simulink model "sampleModel156"  (R2021b)
settings: Solver=VariableStepAuto  StartTime=0.0  StopTime=10.0  RelTol=1e-3
undefined symbols (not defined in the file or in its folder): DiscIntNeverNeededParam, Newton, Raphson
libraries: simulink x12, slpidlib x2
settings Model: Creator=user  LastModifiedBy=user

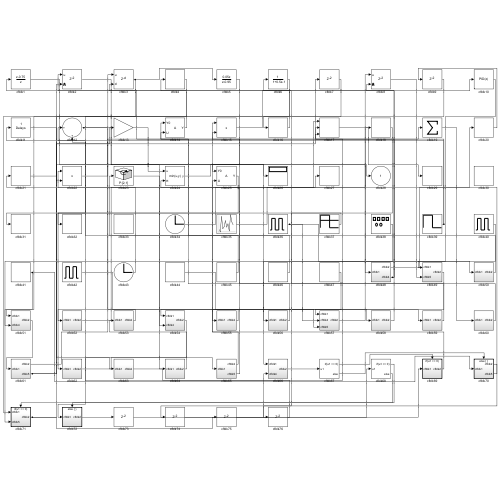
[thumbnail: Simulink's stored preview of the top-level diagram]
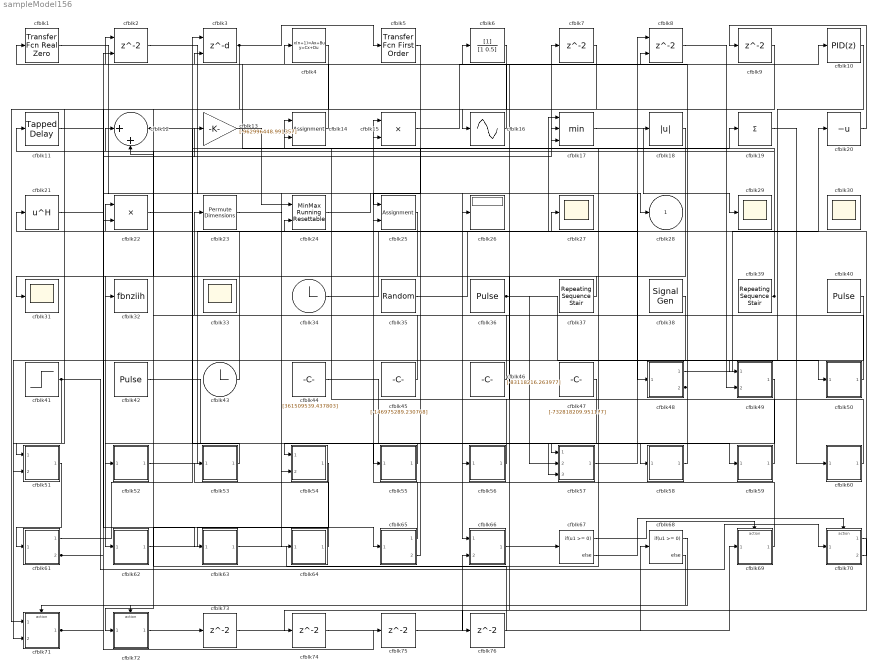
== system sampleModel156 ==
  cfblk1 : simulink/Discrete/Transfer Fcn Real Zero  ZeroZ=0.75  ICPrevInput=0.0  DoSatur=off
      settings: SourceProductBaseCode=SL
  cfblk10 : slpidlib/PID Controller  Controller=PID  Form=Parallel  TimeDomain=Discrete-time  UseExternalTs=off  SampleTime=1  IntegratorMethod=Forward Euler  FilterMethod=Forward Euler  ControllerParametersSource=internal  P=1  I=1  D=0  UseFilter=on  N=100  TunerSelectOption=Transfer Function Based (PID Tuner App)  InitialConditionSource=internal  InitialConditionForIntegrator=0  InitialConditionForFilter=0  DifferentiatorICPrevScaledInput=0  ExternalReset=none  TrackingMode=off  Kt=1  LimitOutput=off  SatLimitsSource=internal  UpperSaturationLimit=inf  LowerSaturationLimit=-inf  LinearizeAsGain=off  AntiWindupMode=none  Kb=1  POutMin=[]  POutMax=[]  IOutMin=[]  IOutMax=[]  DOutMin=[]  DOutMax=[]  NOutMin=[]  NOutMax=[]  SumOutMin=[]  SumOutMax=[]  SaturationOutMin=[]  SaturationOutMax=[]  PParamMin=[]  PParamMax=[]  IParamMin=[]  IParamMax=[]  DParamMin=[]  DParamMax=[]  NParamMin=[]  NParamMax=[]  KbParamMin=[]  KbParamMax=[]  KtParamMin=[]  KtParamMax=[]  KbOutMin=[]  KbOutMax=[]  KtOutMin=[]  KtOutMax=[]  IntegratorOutMin=[]  IntegratorOutMax=[]  FilterOutMin=[]  FilterOutMax=[]  SumI1OutMin=[]  SumI1OutMax=[]  SumI2OutMin=[]  SumI2OutMax=[]  SumI3OutMin=[]  SumI3OutMax=[]  SumI4OutMin=[]  SumI4OutMax=[]  SumDOutMin=[]  SumDOutMax=[]  DifferentiatorOutMin=[]  DifferentiatorOutMax=[]  FilterDiffOutCoefMin=[]  FilterDiffOutCoefMax=[]  ReciprocalOutMin=[]  ReciprocalOutMax=[]  SumDenOutMin=[]  SumDenOutMax=[]  SumNumOutMin=[]  SumNumOutMax=[]  DivideOutMin=[]  DivideOutMax=[]  UdiffTsProdOutMin=[]  UdiffTsProdOutMax=[]  NTsProdOutMin=[]  NTsProdOutMax=[]  UintegralTsProdOutMin=[]  UintegralTsProdOutMax=[]  UngainTsProdOutMin=[]  UngainTsProdOutMax=[]  IntegratorContinuousStateAttributes=''  IntegratorStateMustResolveToSignalObject=off  IntegratorRTWStateStorageClass=Auto  FilterContinuousStateAttributes=''  FilterStateMustResolveToSignalObject=off  FilterRTWStateStorageClass=Auto  ParallelPVariant=InternalParameters  IdealPVariant=Disabled  IVariant=InternalParameters  DVariant=InternalParameters  IntegratorVariant=Discrete  SatVariant=Disabled  AWVariant=Passthrough  PCopyVariant=Disabled  TRVariant=Disabled  FdbkBlocksVariant=Forward  IdealPFdbkVariant=Disabled  SatFdbkVariant=Disabled  DerivativeFilterVariant=ForwardEulerFilter  NVariant=InternalParameters  NCopyVariant=Disabled  FilterICVariant=InternalICsFilter  IntegratorICVariant=InternalICs  ExternalResetVariant=Disabled  TRSumVariant=Passthrough  SumFdbkVariant=Disabled  SumVariant=Sum_PID  TsampFilterVariant=InternalTs  TsampNgainVariant=Passthrough  TsampIntegralVariant=Passthrough  ExternalSaturationOutDataTypeStr=Inherit: Same as second input
  cfblk11 : simulink/Discrete/Tapped Delay  vinit=0.0  samptime=-1  NumDelays=1  DelayOrder=Oldest  includeCurrent=off
  cfblk12 : Sum  Inputs=|++
  cfblk13 : Gain  Gain=[-962996448.991357]
  cfblk14 : Assignment  DiagnosticForDimensions=Warning  IndexOptions=Index vector (dialog)  Indices=1  OutputSizes=1
  cfblk15 : Product  Inputs=**
  cfblk16 : Sin  TimeSource=Use external signal  SampleTime=0
  cfblk17 : MinMax  Inputs=3
  cfblk18 : Abs
  cfblk19 : Sum  Inputs=+
  cfblk2 : Delay  ShowEnablePort=on  SampleTime=1
      settings: InputPortMap=u0,e6
  cfblk20 : UnaryMinus
  cfblk21 : Math  Operator=hermitian  SaturateOnIntegerOverflow=on
  cfblk22 : Product
  cfblk23 : PermuteDimensions
  cfblk24 : simulink/Math Operations/MinMax Running Resettable  Function=min  vinit=0.0
  cfblk25 : Assignment  DiagnosticForDimensions=Warning  IndexOptions=Index vector (dialog)  Indices=1  OutputSizes=1
  cfblk26 : Display
  cfblk{27,29..31,33} (5 alike) : Scope
      cfblk30 settings: Floating=on
      cfblk33 settings: Floating=on
  cfblk3 : Delay  DelayLengthSource=Input port  SampleTime=1
      settings: InputPortMap=u0,p1
  cfblk32 : ToWorkspace  VariableName=fbnziih  SaveFormat=Timeseries  SampleTime=-1
  cfblk34 : Clock
  cfblk35 : UniformRandomNumber  Minimum=[-899286631.365557]  Maximum=[926374637.674813]  Seed=[29961251.000000]  SampleTime=0.1
  cfblk36 : DiscretePulseGenerator  PulseType=Time based  Amplitude=[-229932687.777880]  Period=[45551457.164221]  PulseWidth=5  PhaseDelay=[1.000000]
  cfblk37 : simulink/Sources/Repeating Sequence Stair  OutValues=[272091516.353895, -383976291.141123]  tsamp=-1  OutMin=[]  OutMax=[]  OutDataTypeStr=double  OutputDataTypeScalingMode=double  OutDataType=fixdt(0,8)  ConRadixGroup=Best Precision: Vector-wise  OutScaling=2^-12
  cfblk38 : SignalGenerator  WaveForm=sawtooth  Amplitude=[754582492.273324]
  cfblk39 : simulink/Sources/Repeating Sequence Stair  OutValues=[148032114.325394, 77359554.602000]  tsamp=-1  OutMin=[]  OutMax=[]  OutDataTypeStr=double  OutputDataTypeScalingMode=double  OutDataType=fixdt(0,8)  ConRadixGroup=Best Precision: Vector-wise  OutScaling=2^-12
  cfblk4 : DiscreteStateSpace
  cfblk40 : DiscretePulseGenerator  PulseType=Time based  Amplitude=[574486039.532884]  Period=[50865221.708180]  PulseWidth=5  PhaseDelay=[9.000000]
  cfblk41 : Step  Time=[32.000000]  Before=[271111049.835422]  After=[727022532.262540]  SampleTime=0
  cfblk42 : DiscretePulseGenerator  PulseType=Time based  Amplitude=[-857152997.487512]  Period=[21737191.178487]  PulseWidth=5  PhaseDelay=[9.000000]
  cfblk43 : Clock
  cfblk44 : Constant  Value=[361509539.437803]  SampleTime=1
  cfblk45 : Constant  Value=[-146975289.230768]  SampleTime=1
  cfblk46 : Constant  Value=[-83118216.263977]  SampleTime=1
  cfblk47 : Constant  Value=[-732818209.951177]  SampleTime=1
  cfblk48 : Subsystem
  cfblk49 : Subsystem
  cfblk5 : simulink/Discrete/Transfer Fcn First Order  PoleZ=0.95  ICPrevOutput=0.0  DoSatur=off
  cfblk50 : Subsystem
  cfblk51 : Subsystem
  cfblk52 : Subsystem
  cfblk53 : Subsystem
  cfblk54 : Subsystem
  cfblk55 : Subsystem
  cfblk56 : Subsystem
  cfblk57 : Subsystem
  cfblk58 : Subsystem
  cfblk59 : Subsystem
  cfblk6 : DiscreteFilter  SampleTime=1
  cfblk60 : Subsystem
  cfblk61 : Subsystem
  cfblk62 : Subsystem
  cfblk63 : Subsystem
  cfblk64 : Subsystem
  cfblk65 : Subsystem
  cfblk66 : Subsystem
  cfblk67 : If  IfExpression=u1 >= 0  SampleTime=1
  cfblk68 : If  IfExpression=u1 >= 0  SampleTime=1
  cfblk69 : Subsystem  TreatAsAtomicUnit=on
  cfblk{7,9,73..76} (6 alike) : Delay  SampleTime=1
  cfblk70 : Subsystem  TreatAsAtomicUnit=on
  cfblk71 : Subsystem  TreatAsAtomicUnit=on
  cfblk72 : Subsystem  TreatAsAtomicUnit=on
  cfblk8 : Delay  ShowEnablePort=on  SampleTime=1
      settings: InputPortMap=u0,e6
  cfblk28 : Outport
  wires:
  cfblk65/1(cfblk2) -> cfblk15/1
  cfblk13/1 -> cfblk24/1
  cfblk43/1 -> cfblk22/1
  cfblk51/1(cfblk2) -> cfblk61/1(cfblk1)
  cfblk37/1 -> cfblk31/1
  cfblk17/1 -> cfblk29/1
  cfblk46/1 -> cfblk23/1
  cfblk19/1 -> cfblk60/1(cfblk1)
  cfblk63/1(cfblk2) -> cfblk7/1
  cfblk66/1(cfblk2) -> cfblk67/1
  cfblk22/1 -> cfblk19/1
  cfblk6/1 -> cfblk71/1(cfblk1)
  cfblk48/1(cfblk2) -> cfblk20/1
  cfblk47/1 -> cfblk57/1(cfblk1)
  cfblk2/1 -> cfblk66/1(cfblk1)
  cfblk1/1 -> cfblk64/1(cfblk1)
  cfblk14/1 -> cfblk2/1
  cfblk25/1 -> cfblk62/1(cfblk1)
  cfblk5/1 -> cfblk25/1
  cfblk9/1 -> cfblk16/1
  cfblk65/2(cfblk5) -> cfblk24/2
  cfblk40/1 -> cfblk56/1(cfblk1)
  cfblk39/1 -> cfblk11/1, cfblk3/2
  cfblk36/1 -> cfblk50/1(cfblk1), cfblk57/2(cfblk4)
  cfblk45/1 -> cfblk12/1
  cfblk62/1(cfblk2) -> cfblk65/1(cfblk1)
  cfblk53/1(cfblk2) -> cfblk52/1(cfblk1)
  cfblk38/1 -> cfblk71/2(cfblk5)
  cfblk42/1 -> cfblk58/1(cfblk1)
  cfblk41/1 -> cfblk70/1(cfblk1), cfblk51/2(cfblk4)
  cfblk7/1 -> cfblk51/1(cfblk1)
  cfblk57/1(cfblk2) -> cfblk18/1
  cfblk56/1(cfblk2) -> cfblk14/1
  cfblk3/1 -> cfblk22/2, cfblk5/1
  cfblk35/1 -> cfblk8/1
  cfblk52/1(cfblk2) -> cfblk27/1
  cfblk44/1 -> cfblk59/1(cfblk1)
  cfblk58/1(cfblk2) -> cfblk8/2
  cfblk55/1(cfblk2) -> cfblk54/1(cfblk1)
  cfblk69/1(cfblk2) -> cfblk25/2
  cfblk21/1 -> cfblk26/1
  cfblk59/1(cfblk2) -> cfblk15/2
  cfblk70/2(cfblk5) -> cfblk21/1
  cfblk23/1 -> cfblk54/2(cfblk4)
  cfblk71/1(cfblk2) -> cfblk2/2, cfblk75/1
  cfblk24/1 -> cfblk28/1
  cfblk12/1 -> cfblk48/1(cfblk1), cfblk57/3(cfblk5)
  cfblk15/1 -> cfblk10/1
  cfblk48/2(cfblk4) -> cfblk4/1, cfblk17/3
  cfblk49/1(cfblk2) -> cfblk55/1(cfblk1)
  cfblk61/1(cfblk2) -> cfblk3/1
  cfblk60/1(cfblk2) -> cfblk6/1
  cfblk10/1 -> cfblk49/1(cfblk1)
  cfblk50/1(cfblk2) -> cfblk14/2
  cfblk11/1 -> cfblk63/1(cfblk1)
  cfblk4/1 -> cfblk32/1
  cfblk61/2(cfblk5) -> cfblk13/1, cfblk17/2
  cfblk34/1 -> cfblk17/1
  cfblk20/1 -> cfblk9/1
  cfblk64/1(cfblk2) -> cfblk53/1(cfblk1)
  cfblk54/1(cfblk2) -> cfblk72/1(cfblk1)
  cfblk8/1 -> cfblk49/2(cfblk5)
  cfblk16/1 -> cfblk1/1
  cfblk67/1 -> cfblk69/Action
  cfblk67/2 -> cfblk70/Action
  cfblk68/1 -> cfblk71/Action
  cfblk68/2 -> cfblk72/Action
  cfblk72/1(cfblk2) -> cfblk73/1
  cfblk73/1 -> cfblk69/1(cfblk1)
  cfblk70/1(cfblk2) -> cfblk74/1
  cfblk74/1 -> cfblk66/2(cfblk4)
  cfblk75/1 -> cfblk68/1
  cfblk18/1 -> cfblk76/1
  cfblk76/1 -> cfblk12/2

== system sampleModel156/cfblk48 ==
  cfblk1 : Inport
  cfblk3 : Bias  Bias=[-28596696.417519]
  cfblk2 : Outport
  cfblk4 : Outport  Port=2
  wires:
  cfblk1/1 -> cfblk3/1
  cfblk3/1 -> cfblk2/1, cfblk4/1

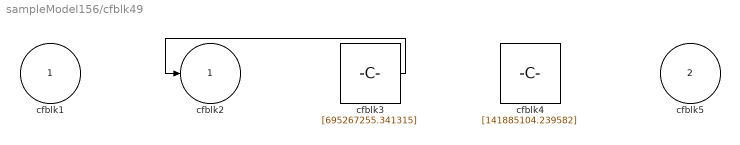
== system sampleModel156/cfblk49 ==
  cfblk1 : Inport
  cfblk5 : Inport  Port=2
  cfblk3 : Constant  Value=[695267255.341315]  SampleTime=1
  cfblk4 : Constant  Value=[141885104.239582]  SampleTime=1
  cfblk2 : Outport
  wires:
  cfblk3/1 -> cfblk2/1

== system sampleModel156/cfblk50 ==
  cfblk1 : Inport
  cfblk3 : Bias  Bias=[731161692.289361]
  cfblk2 : Outport
  wires:
  cfblk1/1 -> cfblk3/1
  cfblk3/1 -> cfblk2/1

== system sampleModel156/cfblk51 ==
  cfblk1 : Inport
  cfblk4 : Inport  Port=2
  cfblk3 : DiscreteFilter  SampleTime=1
  cfblk2 : Outport
  wires:
  cfblk4/1 -> cfblk2/1
  cfblk1/1 -> cfblk3/1

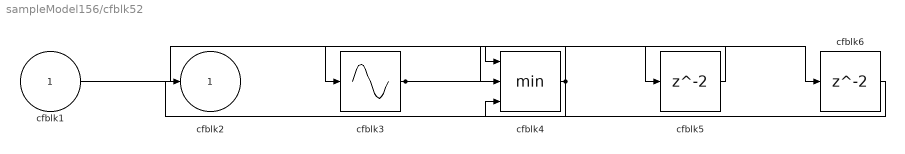
== system sampleModel156/cfblk52 ==
  cfblk1 : Inport
  cfblk3 : Sin  TimeSource=Use external signal  SampleTime=0
  cfblk4 : MinMax  Inputs=3
  cfblk5 : Delay  SampleTime=1
  cfblk6 : Delay  SampleTime=1
  cfblk2 : Outport
  wires:
  cfblk1/1 -> cfblk4/1
  cfblk3/1 -> cfblk5/1, cfblk6/1
  cfblk4/1 -> cfblk2/1, cfblk3/1
  cfblk5/1 -> cfblk4/2
  cfblk6/1 -> cfblk4/3

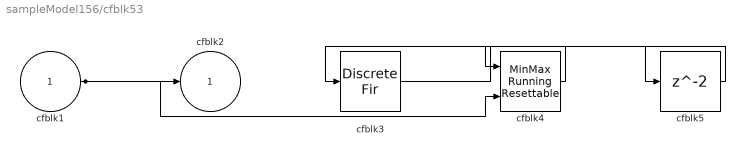
== system sampleModel156/cfblk53 ==
  cfblk1 : Inport
  cfblk3 : DiscreteFir  SampleTime=1
  cfblk4 : simulink/Math Operations/MinMax Running Resettable  Function=min  vinit=0.0
  cfblk5 : Delay  SampleTime=1
  cfblk2 : Outport
  wires:
  cfblk1/1 -> cfblk2/1, cfblk4/2
  cfblk4/1 -> cfblk3/1
  cfblk3/1 -> cfblk5/1
  cfblk5/1 -> cfblk4/1

== system sampleModel156/cfblk54 ==
  cfblk1 : Inport
  cfblk4 : Inport  Port=2
  cfblk3 : Product  Inputs=**
  cfblk2 : Outport
  wires:
  cfblk4/1 -> cfblk3/1
  cfblk1/1 -> cfblk3/2
  cfblk3/1 -> cfblk2/1

== system sampleModel156/cfblk55 ==
  cfblk1 : Inport
  cfblk3 : UnitDelay  HasFrameUpgradeWarning=on
  cfblk4 : Constant  Value=[458405676.200662]  SampleTime=1
  cfblk2 : Outport
  wires:
  cfblk1/1 -> cfblk3/1
  cfblk3/1 -> cfblk2/1

== system sampleModel156/cfblk56 ==
  cfblk1 : Inport
  cfblk3 : Sum  Inputs=+-
  cfblk4 : ComplexToMagnitudeAngle
  cfblk2 : Outport
  wires:
  cfblk4/1 -> cfblk3/1
  cfblk3/1 -> cfblk2/1
  cfblk4/2 -> cfblk3/2
  cfblk1/1 -> cfblk4/1

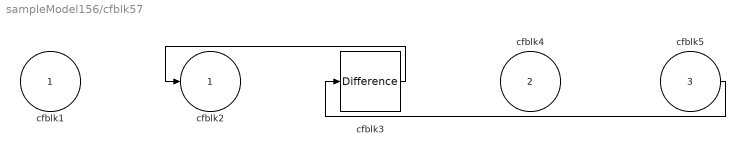
== system sampleModel156/cfblk57 ==
  cfblk1 : Inport
  cfblk4 : Inport  Port=2
  cfblk5 : Inport  Port=3
  cfblk3 : simulink/Discrete/Difference  ICPrevInput=0.0  OutMin=[]  OutMax=[]  OutDataTypeStr=Inherit: Inherit via back propagation  OutDataType=fixdt(1, 16)  OutScaling=2^-10  DoSatur=off
  cfblk2 : Outport
  wires:
  cfblk3/1 -> cfblk2/1
  cfblk5/1 -> cfblk3/1

== system sampleModel156/cfblk58 ==
  cfblk1 : Inport
  cfblk3 : DotProduct  InputSameDT=on  OutDataTypeStr=Inherit: Inherit via internal rule
  cfblk2 : Outport
  wires:
  cfblk1/1 -> cfblk3/1, cfblk3/2
  cfblk3/1 -> cfblk2/1

== system sampleModel156/cfblk59 ==
  cfblk1 : Inport
  cfblk3 : DiscreteStateSpace
  cfblk4 : simulink/Discrete/Transfer Fcn Lead or Lag  PoleZ=0.95  ZeroZ=0.75  ICPrevOutput=0.0  ICPrevInput=0.0  DoSatur=off
      settings: SourceProductBaseCode=SL
  cfblk2 : Outport
  wires:
  cfblk4/1 -> cfblk2/1
  cfblk1/1 -> cfblk3/1
  cfblk3/1 -> cfblk4/1

== system sampleModel156/cfblk60 ==
  cfblk1 : Inport
  cfblk3 : simulink/Discrete/Difference  ICPrevInput=0.0  OutMin=[]  OutMax=[]  OutDataTypeStr=Inherit: Inherit via back propagation  OutDataType=fixdt(1, 16)  OutScaling=2^-10  DoSatur=off
  cfblk4 : Squeeze
  cfblk2 : Outport
  wires:
  cfblk1/1 -> cfblk3/1
  cfblk3/1 -> cfblk4/1
  cfblk4/1 -> cfblk2/1

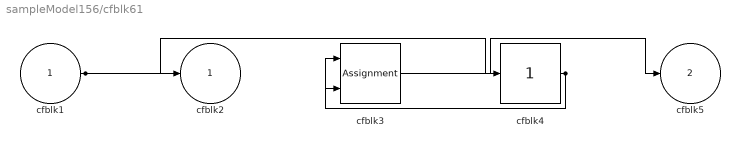
== system sampleModel156/cfblk61 ==
  cfblk1 : Inport
  cfblk3 : Assignment  DiagnosticForDimensions=Warning  IndexOptions=Index vector (dialog)  Indices=1  OutputSizes=1
  cfblk4 : simulink/Math Operations/Slider Gain  gain=1  low=0  high=2
  cfblk2 : Outport
  cfblk5 : Outport  Port=2
  wires:
  cfblk3/1 -> cfblk5/1
  cfblk1/1 -> cfblk2/1, cfblk4/1
  cfblk4/1 -> cfblk3/1, cfblk3/2

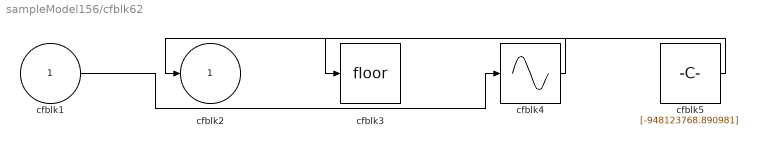
== system sampleModel156/cfblk62 ==
  cfblk1 : Inport
  cfblk3 : Rounding
  cfblk4 : Sin  TimeSource=Use external signal  SampleTime=0
  cfblk5 : Constant  Value=[-948123768.890981]  SampleTime=1
  cfblk2 : Outport
  wires:
  cfblk4/1 -> cfblk2/1
  cfblk1/1 -> cfblk4/1
  cfblk5/1 -> cfblk3/1

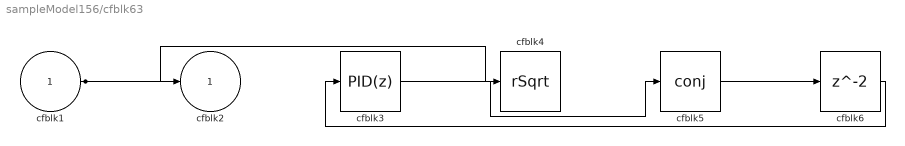
== system sampleModel156/cfblk63 ==
  cfblk1 : Inport
  cfblk3 : slpidlib/PID Controller  Controller=PID  Form=Parallel  TimeDomain=Discrete-time  UseExternalTs=off  SampleTime=1  IntegratorMethod=Forward Euler  FilterMethod=Forward Euler  ControllerParametersSource=internal  P=1  I=1  D=0  UseFilter=on  N=100  TunerSelectOption=Transfer Function Based (PID Tuner App)  InitialConditionSource=internal  InitialConditionForIntegrator=0  InitialConditionForFilter=0  DifferentiatorICPrevScaledInput=0  ExternalReset=none  TrackingMode=off  Kt=1  LimitOutput=off  SatLimitsSource=internal  UpperSaturationLimit=inf  LowerSaturationLimit=-inf  LinearizeAsGain=off  AntiWindupMode=none  Kb=1  POutMin=[]  POutMax=[]  IOutMin=[]  IOutMax=[]  DOutMin=[]  DOutMax=[]  NOutMin=[]  NOutMax=[]  SumOutMin=[]  SumOutMax=[]  SaturationOutMin=[]  SaturationOutMax=[]  PParamMin=[]  PParamMax=[]  IParamMin=[]  IParamMax=[]  DParamMin=[]  DParamMax=[]  NParamMin=[]  NParamMax=[]  KbParamMin=[]  KbParamMax=[]  KtParamMin=[]  KtParamMax=[]  KbOutMin=[]  KbOutMax=[]  KtOutMin=[]  KtOutMax=[]  IntegratorOutMin=[]  IntegratorOutMax=[]  FilterOutMin=[]  FilterOutMax=[]  SumI1OutMin=[]  SumI1OutMax=[]  SumI2OutMin=[]  SumI2OutMax=[]  SumI3OutMin=[]  SumI3OutMax=[]  SumI4OutMin=[]  SumI4OutMax=[]  SumDOutMin=[]  SumDOutMax=[]  DifferentiatorOutMin=[]  DifferentiatorOutMax=[]  FilterDiffOutCoefMin=[]  FilterDiffOutCoefMax=[]  ReciprocalOutMin=[]  ReciprocalOutMax=[]  SumDenOutMin=[]  SumDenOutMax=[]  SumNumOutMin=[]  SumNumOutMax=[]  DivideOutMin=[]  DivideOutMax=[]  UdiffTsProdOutMin=[]  UdiffTsProdOutMax=[]  NTsProdOutMin=[]  NTsProdOutMax=[]  UintegralTsProdOutMin=[]  UintegralTsProdOutMax=[]  UngainTsProdOutMin=[]  UngainTsProdOutMax=[]  IntegratorContinuousStateAttributes=''  IntegratorStateMustResolveToSignalObject=off  IntegratorRTWStateStorageClass=Auto  FilterContinuousStateAttributes=''  FilterStateMustResolveToSignalObject=off  FilterRTWStateStorageClass=Auto  ParallelPVariant=InternalParameters  IdealPVariant=Disabled  IVariant=InternalParameters  DVariant=InternalParameters  IntegratorVariant=Discrete  SatVariant=Disabled  AWVariant=Passthrough  PCopyVariant=Disabled  TRVariant=Disabled  FdbkBlocksVariant=Forward  IdealPFdbkVariant=Disabled  SatFdbkVariant=Disabled  DerivativeFilterVariant=ForwardEulerFilter  NVariant=InternalParameters  NCopyVariant=Disabled  FilterICVariant=InternalICsFilter  IntegratorICVariant=InternalICs  ExternalResetVariant=Disabled  TRSumVariant=Passthrough  SumFdbkVariant=Disabled  SumVariant=Sum_PID  TsampFilterVariant=InternalTs  TsampNgainVariant=Passthrough  TsampIntegralVariant=Passthrough  ExternalSaturationOutDataTypeStr=Inherit: Same as second input
  cfblk4 : Sqrt  Operator=rSqrt  AlgorithmType=Newton-Raphson  SaturateOnIntegerOverflow=on
  cfblk5 : Math  Operator=conj  SaturateOnIntegerOverflow=on
  cfblk6 : Delay  SampleTime=1
  cfblk2 : Outport
  wires:
  cfblk1/1 -> cfblk2/1, cfblk4/1
  cfblk3/1 -> cfblk5/1
  cfblk5/1 -> cfblk6/1
  cfblk6/1 -> cfblk3/1

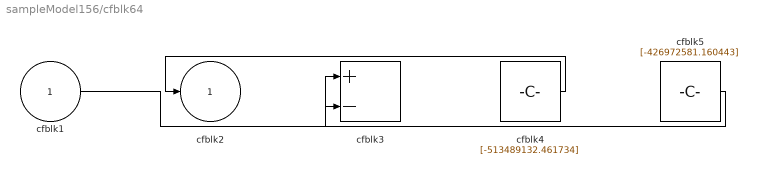
== system sampleModel156/cfblk64 ==
  cfblk1 : Inport
  cfblk3 : Sum  Inputs=+-
  cfblk4 : Constant  Value=[-513489132.461734]  SampleTime=1
  cfblk5 : Constant  Value=[-426972581.160443]  SampleTime=1
  cfblk2 : Outport
  wires:
  cfblk4/1 -> cfblk2/1
  cfblk5/1 -> cfblk3/1
  cfblk1/1 -> cfblk3/2

== system sampleModel156/cfblk65 ==
  cfblk1 : Inport
  cfblk3 : Reshape
  cfblk4 : Sum  Inputs=+
  cfblk2 : Outport
  cfblk5 : Outport  Port=2
  wires:
  cfblk4/1 -> cfblk3/1
  cfblk3/1 -> cfblk5/1
  cfblk1/1 -> cfblk2/1, cfblk4/1

== system sampleModel156/cfblk66 ==
  cfblk1 : Inport
  cfblk4 : Inport  Port=2
  cfblk3 : MinMax
  cfblk2 : Outport
  wires:
  cfblk1/1 -> cfblk3/1
  cfblk4/1 -> cfblk2/1

== system sampleModel156/cfblk69 ==
  cfblk1 : Inport
  Action Port : ActionPort  ActionPortLabel=if(u1 >= 0)
  cfblk3 : DiscreteIntegrator  SampleTime=-1  ICPrevOutput=DiscIntNeverNeededParam  ICPrevScaledInput=DiscIntNeverNeededParam
  cfblk2 : Outport
  wires:
  cfblk1/1 -> cfblk2/1, cfblk3/1

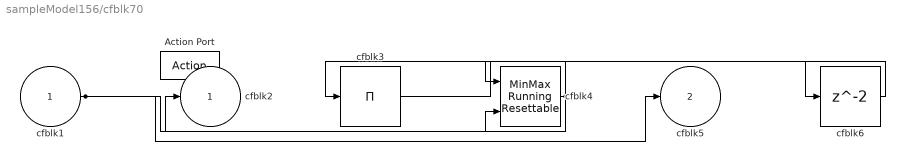
== system sampleModel156/cfblk70 ==
  cfblk1 : Inport
  Action Port : ActionPort  ActionPortLabel=else
  cfblk3 : Product  Inputs=*
  cfblk4 : simulink/Math Operations/MinMax Running Resettable  Function=min  vinit=0.0
  cfblk6 : Delay
  cfblk2 : Outport
  cfblk5 : Outport  Port=2
  wires:
  cfblk4/1 -> cfblk2/1, cfblk3/1
  cfblk1/1 -> cfblk5/1, cfblk4/2
  cfblk3/1 -> cfblk6/1
  cfblk6/1 -> cfblk4/1

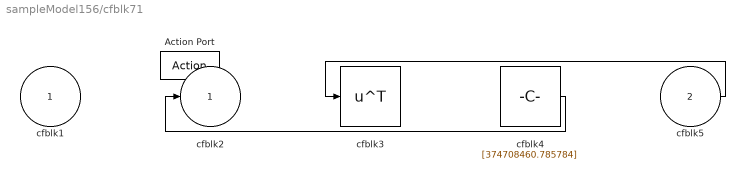
== system sampleModel156/cfblk71 ==
  cfblk1 : Inport
  cfblk5 : Inport  Port=2
  Action Port : ActionPort  ActionPortLabel=if(u1 >= 0)
  cfblk3 : Math  Operator=transpose  SaturateOnIntegerOverflow=on
  cfblk4 : Constant  Value=[374708460.785784]  SampleTime=1
  cfblk2 : Outport
  wires:
  cfblk4/1 -> cfblk2/1
  cfblk5/1 -> cfblk3/1

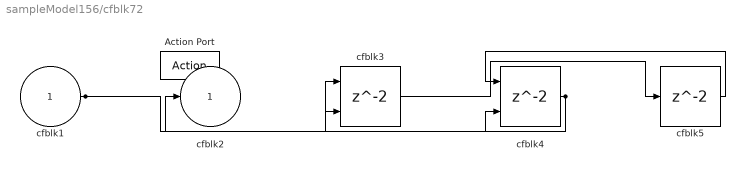
== system sampleModel156/cfblk72 ==
  cfblk1 : Inport
  Action Port : ActionPort  ActionPortLabel=else
  cfblk3 : Delay  ShowEnablePort=on
      settings: InputPortMap=u0,e6
  cfblk4 : Delay  ShowEnablePort=on
      settings: InputPortMap=u0,e6
  cfblk5 : Delay
  cfblk2 : Outport
  wires:
  cfblk4/1 -> cfblk2/1, cfblk3/2
  cfblk1/1 -> cfblk4/2, cfblk3/1
  cfblk3/1 -> cfblk5/1
  cfblk5/1 -> cfblk4/1
